simulink model "phase4_scheduler_application"  (R2026a)
settings: Solver=FixedStepDiscrete  EnableMultiTasking=on
undefined symbols (not defined in the file): CostWeights, MapMaximumNearestDistance, MapNormalizationMean, MapNormalizationScale, MapRawMaximum, MapRawMinimum, MapSafetyMargins, MapSampleTimes_s, MapX, MapY, MaximumCpuUtilization, MaximumHeadingError_rad, MaximumLateralError_m, ModeCpuAdmissible, ModeMeanCpuUtilization, phase4_scheduler_application
libraries: proctasklib x1
settings Model: Creator=The MathWorks, Inc.  LastModifiedBy=rayyu
settings SolverCC: PositivePriorityOrder=on
settings HardwareCC: ProdBitPerLong=64.0  ProdLargestAtomicInteger=LongLong  ProdLargestAtomicFloat=Double  ProdHWDeviceType=ARM Compatible->ARM Cortex-A (64-bit)  HardwareBoardFeatureSet=SoCBlockset
settings RTWCC: SystemTargetFile=ert.tlc  HardwareBoard=Xilinx Zynq UltraScale+ MPSoC ZCU102 Evaluation Kit  TLCOptions="-aInlineSetEventsForThisBaseRateFcn=TLC_FALSE -aSuppressMultiTaskScheduler=TLC_FALSE  -aRateBasedStepFcn=0"  GenerateReport=on  Toolchain=Linaro AArch64 Linux v6.3.1  IncludeHyperlinkInReport=on  LaunchReport=on  GenerateTraceInfo=on  GenerateTraceReport=on  GenerateTraceReportSl=on  GenerateTraceReportSf=on  GenerateTraceReportEml=on  Description=Embedded Coder
settings ERTTargetCC: ExtModeTransport=2.0  DynamicArrayContainerType=coder::array

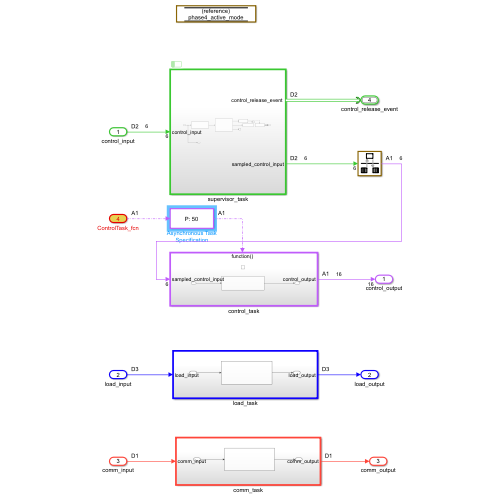
[thumbnail: Simulink's stored preview of the top-level diagram]
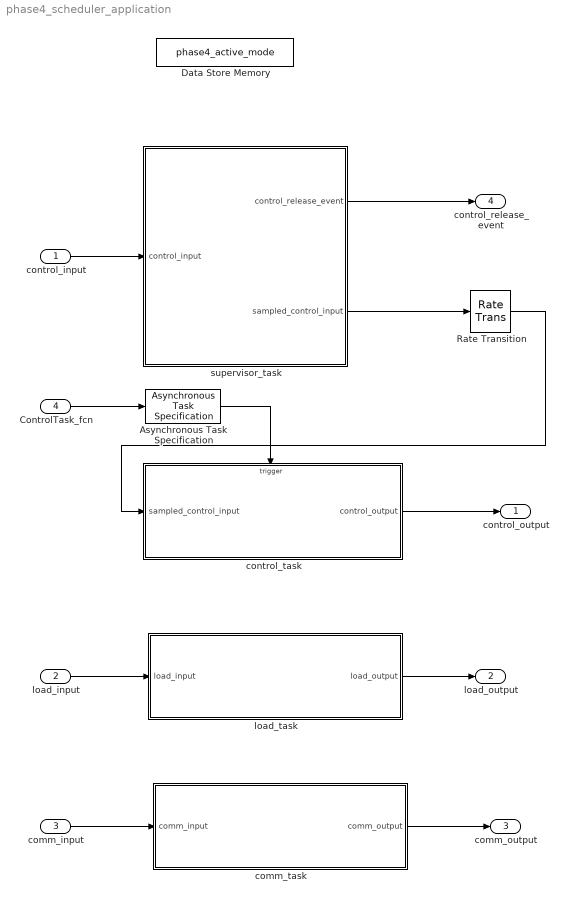
== system phase4_scheduler_application ==
  control_input : Inport
  load_input : Inport  Port=2  SampleTime=0.05  Interpolate=off
  comm_input : Inport  Port=3  SampleTime=0.005  Interpolate=off
  ControlTask_fcn : Inport  Port=4  OutputFunctionCall=on
  Asynchronous Task Specification : AsynchronousTaskSpecification  TaskPriority=50
  Data Store Memory : DataStoreMemory  DataStoreName=phase4_active_mode  WriteAfterWriteMsg=warning  DataStoreReference=on  ShowAdditionalParam=off  OutDataTypeStr=uint8  Dimensions=1
  Rate Transition : RateTransition  Deterministic=off
  comm_task : Subsystem  TreatAsAtomicUnit=on
  control_task : Subsystem  TreatAsAtomicUnit=on
  load_task : Subsystem  TreatAsAtomicUnit=on
  supervisor_task : Subsystem  TreatAsAtomicUnit=on  ScheduleAs=Periodic partition  PartitionName=SupervisorTask  SystemSampleTime=0.01
  control_output : Outport  VectorParamsAs1DForOutWhenUnconnected=off
  load_output : Outport  Port=2  VectorParamsAs1DForOutWhenUnconnected=off
  comm_output : Outport  Port=3
  control_release_event : Outport  InputPortMessageModes=m  Port=4  OutDataTypeStr=Bus: rteEvent  BusOutputAsStruct=on
  wires:
  control_task/1(control_output) -> control_output/1
  control_input/1 -> supervisor_task/1(control_input)
  load_input/1 -> load_task/1(load_input)
  load_task/1(load_output) -> load_output/1
  comm_input/1 -> comm_task/1(comm_input)
  comm_task/1(comm_output) -> comm_output/1
  supervisor_task/1("control_release_event ") -> control_release_event/1
  ControlTask_fcn/1 -> Asynchronous Task Specification/1
  Asynchronous Task Specification/1 -> control_task/Trigger
  supervisor_task/2(sampled_control_input) -> Rate Transition/1
  Rate Transition/1 -> control_task/1(sampled_control_input)

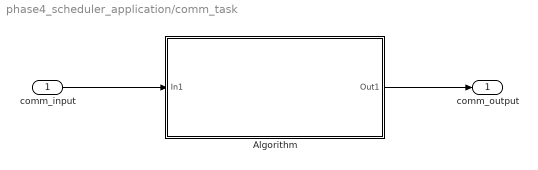
== system phase4_scheduler_application/comm_task ==
  comm_input : Inport
  Algorithm : Subsystem
  comm_output : Outport  VectorParamsAs1DForOutWhenUnconnected=off
  wires:
  comm_input/1 -> Algorithm/1(In1)
  Algorithm/1(Out1) -> comm_output/1

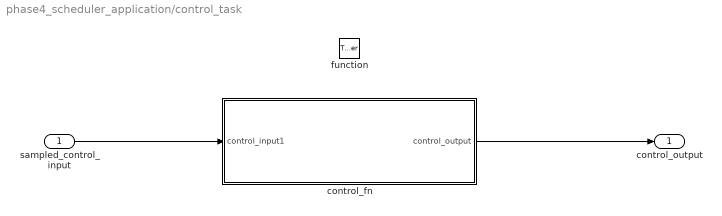
== system phase4_scheduler_application/control_task ==
  sampled_control_input : Inport
  function : TriggerPort  TriggerType=function-call  VariantControl=(inherit)
  control_fn : Subsystem  TreatAsAtomicUnit=on
  control_output : Outport
  wires:
  sampled_control_input/1 -> control_fn/1(control_input1)
  control_fn/1(control_output) -> control_output/1

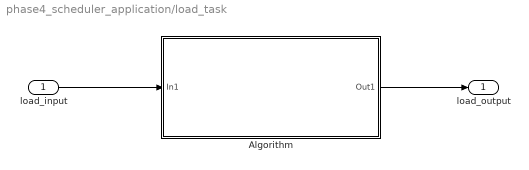
== system phase4_scheduler_application/load_task ==
  load_input : Inport
  Algorithm : Subsystem
  load_output : Outport  VectorParamsAs1DForOutWhenUnconnected=off
  wires:
  Algorithm/1(Out1) -> load_output/1
  load_input/1 -> Algorithm/1(In1)

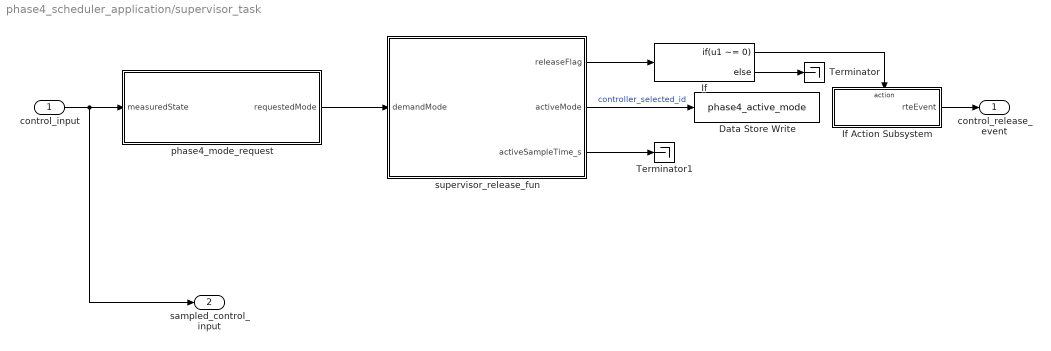
== system phase4_scheduler_application/supervisor_task ==
  control_input : Inport
  Data Store Write : DataStoreWrite  DataStoreName=phase4_active_mode  IndexOptions=Index vector (dialog)  Indices=1  OutputSizes=1
  If : If  IfExpression=u1 ~= 0
  If Action Subsystem : Subsystem  TreatAsAtomicUnit=on
  Terminator : Terminator
  Terminator1 : Terminator
  phase4_mode_request : Subsystem
  supervisor_release_fun : MATLAB Function  TreatAsAtomicUnit=on
  "control_release_event " : Outport  OutDataTypeStr=Bus: rteEvent
  sampled_control_input : Outport  Port=2
  wires:
  supervisor_release_fun/1(releaseFlag) -> If/1
  supervisor_release_fun/2(activeMode) -> Data Store Write/1  "controller_selected_id"
  supervisor_release_fun/3(activeSampleTime_s) -> Terminator1/1
  If/1 -> If Action Subsystem/Action
  If/2 -> Terminator/1
  If Action Subsystem/1(rteEvent) -> "control_release_event "/1
  phase4_mode_request/1(requestedMode) -> supervisor_release_fun/1(demandMode)
  control_input/1 -> sampled_control_input/1, phase4_mode_request/1(measuredState)

== system phase4_scheduler_application/comm_task/Algorithm ==
  In1 : Inport
  Gain : Gain  Gain=-1
  Out1 : Outport  VectorParamsAs1DForOutWhenUnconnected=off
  wires:
  Gain/1 -> Out1/1
  In1/1 -> Gain/1

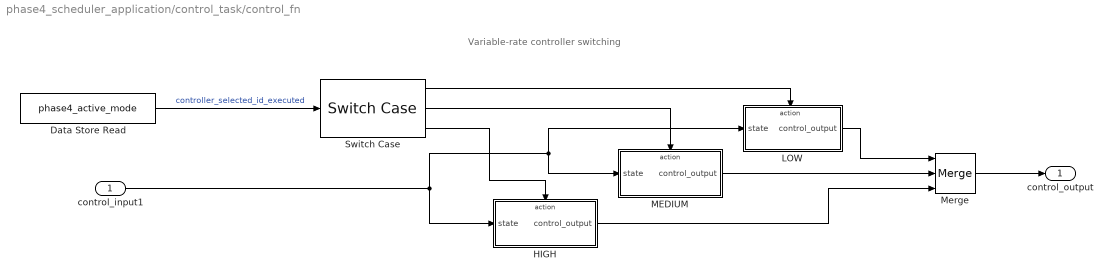
== system phase4_scheduler_application/control_task/control_fn ==
  note: Variable-rate controller switching
  control_input1 : Inport
  Data Store Read : DataStoreRead  DataStoreName=phase4_active_mode  IndexOptions=Index vector (dialog)  Indices=1  OutputSizes=1
  HIGH : Subsystem  TreatAsAtomicUnit=on
  LOW : Subsystem  TreatAsAtomicUnit=on
  MEDIUM : Subsystem  TreatAsAtomicUnit=on
  Merge : Merge  Inputs=3
  Switch Case : SwitchCase  CaseConditions={1, 2, 3}  ShowDefaultCase=off
  control_output : Outport
  wires:
  control_input1/1 -> HIGH/1(state), LOW/1(state), MEDIUM/1(state)
  Data Store Read/1 -> Switch Case/1  "controller_selected_id_executed"
  Switch Case/1 -> LOW/Action
  Switch Case/2 -> MEDIUM/Action
  Switch Case/3 -> HIGH/Action
  LOW/1(control_output) -> Merge/1
  MEDIUM/1(control_output) -> Merge/2
  HIGH/1(control_output) -> Merge/3
  Merge/1 -> control_output/1

== system phase4_scheduler_application/load_task/Algorithm ==
  In1 : Inport
  Gain : Gain  Gain=-1
  Out1 : Outport  VectorParamsAs1DForOutWhenUnconnected=off
  wires:
  In1/1 -> Gain/1
  Gain/1 -> Out1/1

== system phase4_scheduler_application/supervisor_task/If Action Subsystem ==
  Action Port : ActionPort  ActionPortLabel=if(u1 ~= 0)
  Task Trigger : proctasklib/Task Trigger  BlockSID=phase4_scheduler_application:90
  rteEvent : Outport
  wires:
  Task Trigger/1 -> rteEvent/1

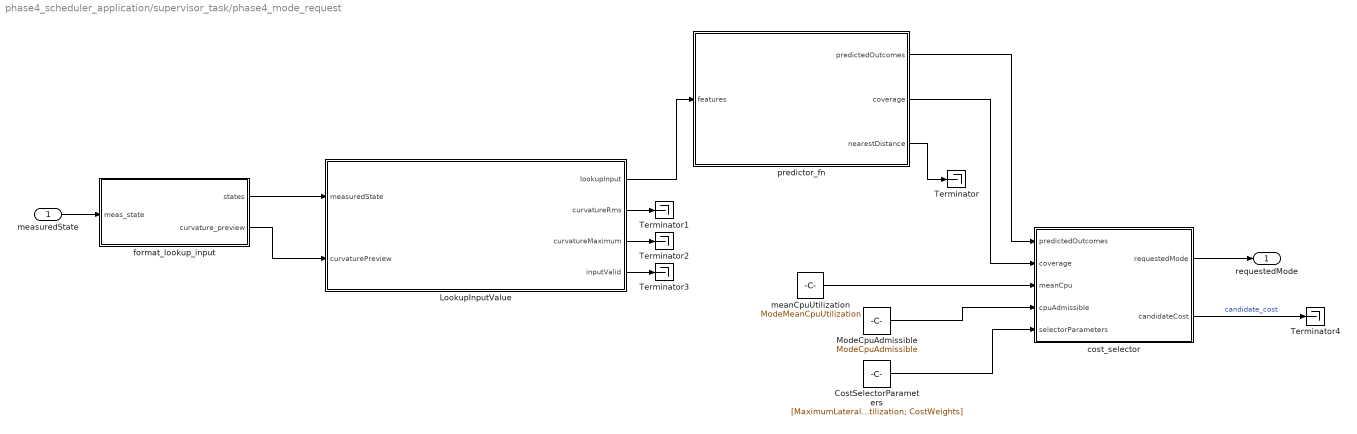
== system phase4_scheduler_application/supervisor_task/phase4_mode_request ==
  measuredState : Inport
  CostSelectorParameters : Constant  Value=[MaximumLateralError_m; MaximumHeadingError_rad; MaximumCpuUtilization; CostWeights]
  LookupInputValue : MATLAB Function  TreatAsAtomicUnit=on
  ModeCpuAdmissible : Constant  Value=ModeCpuAdmissible
  Terminator{,1..4} (5 alike) : Terminator
  cost_selector : MATLAB Function  TreatAsAtomicUnit=on
  format_lookup_input : Subsystem
  meanCpuUtilization : Constant  Value=ModeMeanCpuUtilization
  predictor_fn : MATLAB Function  TreatAsAtomicUnit=on
  requestedMode : Outport
  wires:
  LookupInputValue/1(lookupInput) -> predictor_fn/1(features)
  measuredState/1 -> format_lookup_input/1(meas_state)
  format_lookup_input/1(states) -> LookupInputValue/1(measuredState)
  format_lookup_input/2(curvature_preview) -> LookupInputValue/2(curvaturePreview)
  predictor_fn/1(predictedOutcomes) -> cost_selector/1(predictedOutcomes)
  predictor_fn/2(coverage) -> cost_selector/2(coverage)
  meanCpuUtilization/1 -> cost_selector/3(meanCpu)
  ModeCpuAdmissible/1 -> cost_selector/4(cpuAdmissible)
  CostSelectorParameters/1 -> cost_selector/5(selectorParameters)
  cost_selector/1(requestedMode) -> requestedMode/1
  predictor_fn/3(nearestDistance) -> Terminator/1
  LookupInputValue/2(curvatureRms) -> Terminator1/1
  LookupInputValue/3(curvatureMaximum) -> Terminator2/1
  LookupInputValue/4(inputValid) -> Terminator3/1
  cost_selector/2(candidateCost) -> Terminator4/1  "candidate_cost"

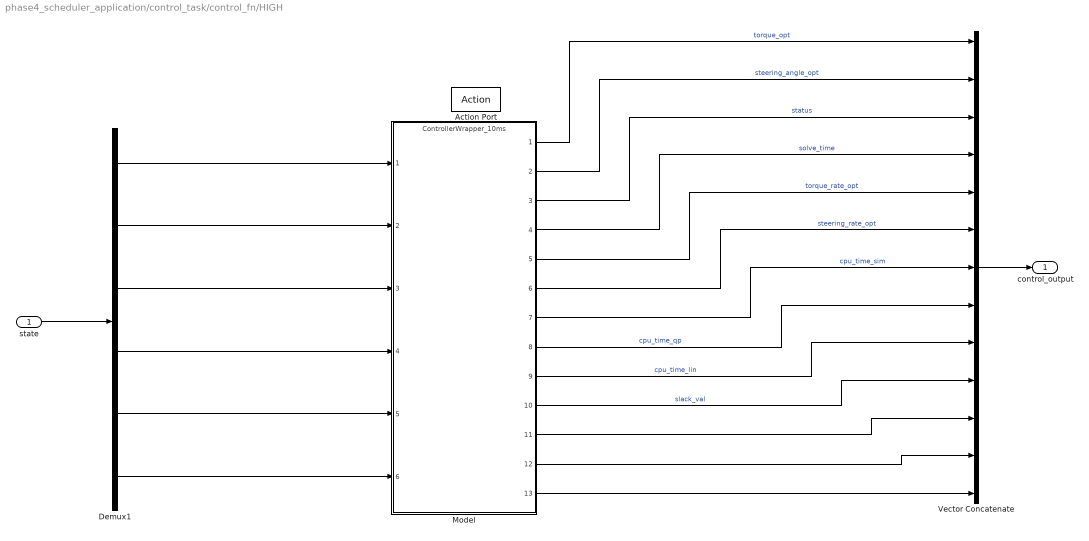
== system phase4_scheduler_application/control_task/control_fn/HIGH ==
  state : Inport
  Action Port : ActionPort  ActionPortLabel=case [ 3 ]:
  Demux1 : Demux  Outputs=6
  Model : ModelReference  ModelNameDialog=ControllerWrapper_10ms.slx  SimulationMode=Normal  ModelReferenceVersion=1.55
  Vector Concatenate : Concatenate  NumInputs=13
  control_output : Outport
  wires:
  Demux1/3 -> Model/3
  Demux1/2 -> Model/2
  Demux1/6 -> Model/6
  Demux1/1 -> Model/1
  state/1 -> Demux1/1
  Demux1/5 -> Model/5
  Demux1/4 -> Model/4
  Model/4 -> Vector Concatenate/4  "solve_time"
  Model/10 -> Vector Concatenate/10  "slack_val"
  Model/3 -> Vector Concatenate/3  "status"
  Model/8 -> Vector Concatenate/8  "cpu_time_qp"
  Model/1 -> Vector Concatenate/1  "torque_opt"
  Model/6 -> Vector Concatenate/6  "steering_rate_opt"
  Vector Concatenate/1 -> control_output/1
  Model/9 -> Vector Concatenate/9  "cpu_time_lin"
  Model/7 -> Vector Concatenate/7  "cpu_time_sim"
  Model/2 -> Vector Concatenate/2  "steering_angle_opt"
  Model/5 -> Vector Concatenate/5  "torque_rate_opt"
  Model/11 -> Vector Concatenate/11
  Model/12 -> Vector Concatenate/12
  Model/13 -> Vector Concatenate/13

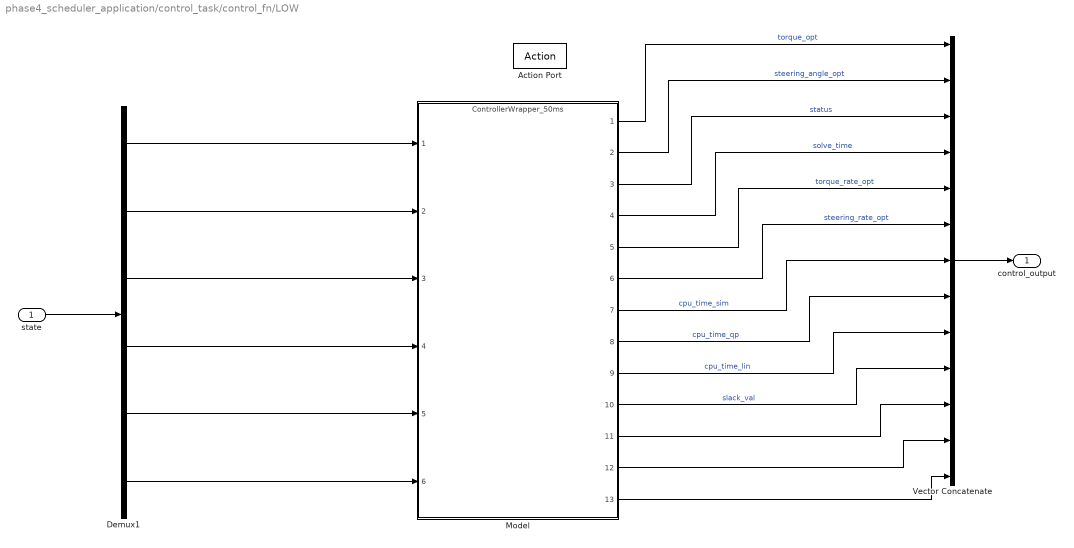
== system phase4_scheduler_application/control_task/control_fn/LOW ==
  state : Inport
  Action Port : ActionPort  ActionPortLabel=case [ 1 ]:
  Demux1 : Demux  Outputs=6
  Model : ModelReference  ModelNameDialog=ControllerWrapper_50ms.slx  SimulationMode=Normal  ModelReferenceVersion=1.51
  Vector Concatenate : Concatenate  NumInputs=13
  control_output : Outport
  wires:
  Demux1/3 -> Model/3
  Demux1/2 -> Model/2
  Demux1/6 -> Model/6
  Demux1/1 -> Model/1
  state/1 -> Demux1/1
  Demux1/5 -> Model/5
  Demux1/4 -> Model/4
  Model/4 -> Vector Concatenate/4  "solve_time"
  Model/10 -> Vector Concatenate/10  "slack_val"
  Model/3 -> Vector Concatenate/3  "status"
  Model/8 -> Vector Concatenate/8  "cpu_time_qp"
  Model/1 -> Vector Concatenate/1  "torque_opt"
  Model/6 -> Vector Concatenate/6  "steering_rate_opt"
  Vector Concatenate/1 -> control_output/1
  Model/9 -> Vector Concatenate/9  "cpu_time_lin"
  Model/7 -> Vector Concatenate/7  "cpu_time_sim"
  Model/2 -> Vector Concatenate/2  "steering_angle_opt"
  Model/5 -> Vector Concatenate/5  "torque_rate_opt"
  Model/11 -> Vector Concatenate/11
  Model/12 -> Vector Concatenate/12
  Model/13 -> Vector Concatenate/13

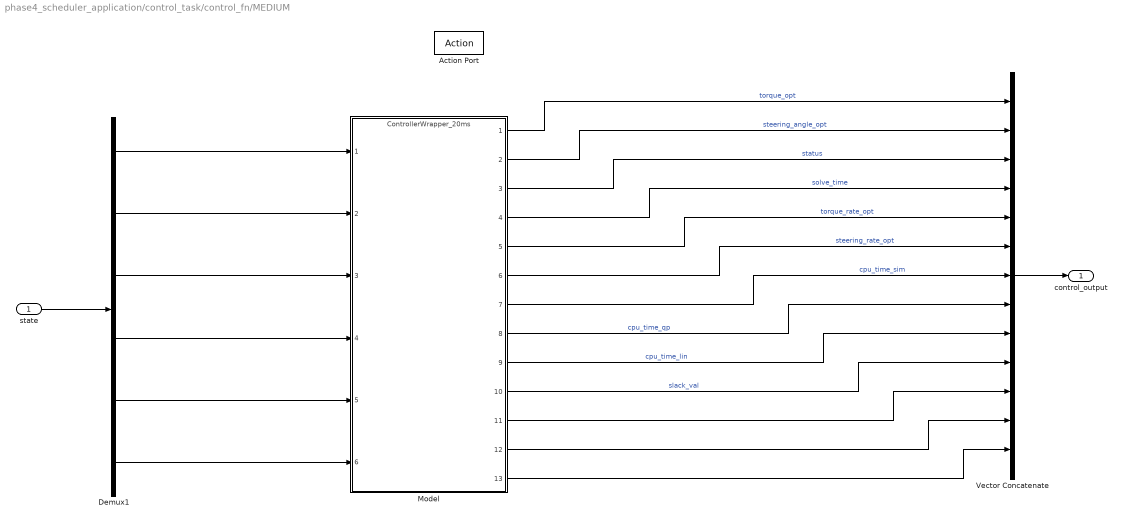
== system phase4_scheduler_application/control_task/control_fn/MEDIUM ==
  state : Inport
  Action Port : ActionPort  ActionPortLabel=case [ 2 ]:
  Demux1 : Demux  Outputs=6
  Model : ModelReference  ModelNameDialog=ControllerWrapper_20ms.slx  SimulationMode=Normal  ModelReferenceVersion=1.53
  Vector Concatenate : Concatenate  NumInputs=13
  control_output : Outport
  wires:
  Demux1/3 -> Model/3
  Demux1/2 -> Model/2
  Demux1/6 -> Model/6
  Demux1/1 -> Model/1
  state/1 -> Demux1/1
  Demux1/5 -> Model/5
  Demux1/4 -> Model/4
  Model/3 -> Vector Concatenate/3  "status"
  Model/4 -> Vector Concatenate/4  "solve_time"
  Model/2 -> Vector Concatenate/2  "steering_angle_opt"
  Model/1 -> Vector Concatenate/1  "torque_opt"
  Vector Concatenate/1 -> control_output/1
  Model/5 -> Vector Concatenate/5  "torque_rate_opt"
  Model/6 -> Vector Concatenate/6  "steering_rate_opt"
  Model/7 -> Vector Concatenate/7  "cpu_time_sim"
  Model/8 -> Vector Concatenate/8  "cpu_time_qp"
  Model/9 -> Vector Concatenate/9  "cpu_time_lin"
  Model/10 -> Vector Concatenate/10  "slack_val"
  Model/11 -> Vector Concatenate/11
  Model/12 -> Vector Concatenate/12
  Model/13 -> Vector Concatenate/13

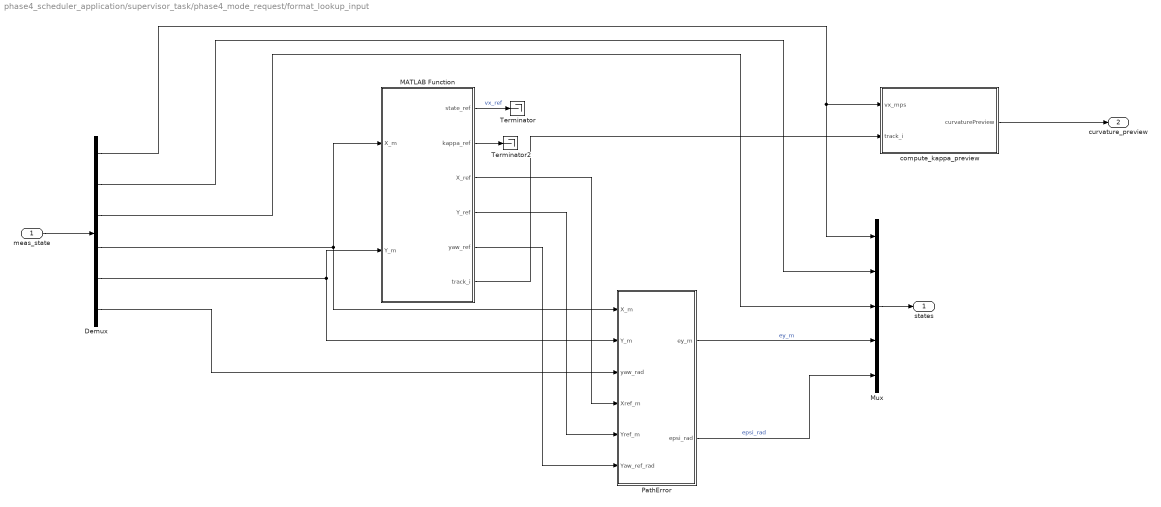
== system phase4_scheduler_application/supervisor_task/phase4_mode_request/format_lookup_input ==
  meas_state : Inport
  Demux : Demux  Outputs=6
  MATLAB Function : MATLAB Function  TreatAsAtomicUnit=on
  Mux : Mux  Inputs=5
  PathError : Subsystem
  Terminator : Terminator
  Terminator2 : Terminator
  compute_kappa_preview : MATLAB Function  TreatAsAtomicUnit=on
  states : Outport
  curvature_preview : Outport  Port=2
  wires:
  MATLAB Function/1(state_ref) -> Terminator/1  "vx_ref"
  MATLAB Function/2(kappa_ref) -> Terminator2/1
  MATLAB Function/3(X_ref) -> PathError/4(Xref_m)
  MATLAB Function/4(Y_ref) -> PathError/5(Yref_m)
  MATLAB Function/5(yaw_ref) -> PathError/6(Yaw_ref_rad)
  MATLAB Function/6(track_i) -> compute_kappa_preview/2(track_i)
  Demux/4 -> PathError/1(X_m), MATLAB Function/1(X_m)
  Demux/5 -> PathError/2(Y_m), MATLAB Function/2(Y_m)
  Demux/6 -> PathError/3(yaw_rad)
  PathError/1(ey_m) -> Mux/4  "ey_m"
  PathError/2(epsi_rad) -> Mux/5  "epsi_rad"
  meas_state/1 -> Demux/1
  Demux/1 -> Mux/1, compute_kappa_preview/1(vx_mps)
  Demux/2 -> Mux/2
  Demux/3 -> Mux/3
  Mux/1 -> states/1
  compute_kappa_preview/1(curvaturePreview) -> curvature_preview/1

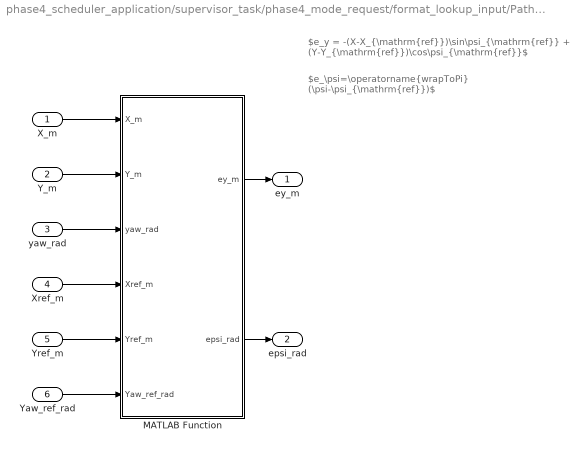
== system phase4_scheduler_application/supervisor_task/phase4_mode_request/format_lookup_input/PathError ==
  note: $e_\psi=\operatorname{wrapToPi} (\psi-\psi_{\mathrm{ref}})$
  note: $e_y = -(X-X_{\mathrm{ref}})\sin\psi_{\mathrm{ref}} + (Y-Y_{\mathrm{ref}})\cos\psi_{\mathrm{ref}}$
  X_m : Inport
  Y_m : Inport  Port=2
  yaw_rad : Inport  Port=3
  Xref_m : Inport  Port=4
  Yref_m : Inport  Port=5
  Yaw_ref_rad : Inport  Port=6
  MATLAB Function : MATLAB Function  TreatAsAtomicUnit=on
  ey_m : Outport
  epsi_rad : Outport  Port=2
  wires:
  X_m/1 -> MATLAB Function/1(X_m)
  Y_m/1 -> MATLAB Function/2(Y_m)
  yaw_rad/1 -> MATLAB Function/3(yaw_rad)
  Xref_m/1 -> MATLAB Function/4(Xref_m)
  Yref_m/1 -> MATLAB Function/5(Yref_m)
  Yaw_ref_rad/1 -> MATLAB Function/6(Yaw_ref_rad)
  MATLAB Function/1(ey_m) -> ey_m/1
  MATLAB Function/2(epsi_rad) -> epsi_rad/1

== matlab function phase4_scheduler_application/supervisor_task/phase4_mode_request/predictor_fn ==
  data: features input double size=[7 1]; predictedOutcomes output double size=[3 6]; coverage output boolean size=[3 1]; nearestDistance output double size=[3 1]; MapRawMaximum parameter size=[3 7]; MapX parameter size=[1146 7]; MapY parameter size=[1146 6]; MapSampleTimes_s parameter size=[1146 1]; MapNormalizationMean parameter size=[1 7]; MapNormalizationScale parameter size=[1 7]; MapRawMinimum parameter size=[3 7]; MapSafetyMargins parameter size=[1 6]; MapMaximumNearestDistance parameter size=[3 1]
function [predictedOutcomes, coverage, nearestDistance] = ...
    lookupPredictor(features, MapRawMaximum, MapX, MapY, MapSampleTimes_s, MapNormalizationMean, MapNormalizationScale, MapRawMinimum, MapSafetyMargins, MapMaximumNearestDistance)

candidateSampleTimes_s = [
    0.050
    0.020
    0.010
    ];

[predictedOutcomes, coverage, nearestDistance] = ...
    sdv.supervisor.predictFromLookupMap( ...
        features, ...
        candidateSampleTimes_s, ...
        MapX, ...
        MapY, ...
        MapSampleTimes_s, ...
        MapNormalizationMean, ...
        MapNormalizationScale, ...
        MapRawMinimum, ...
        MapRawMaximum, ...
        MapSafetyMargins, ...
        MapMaximumNearestDistance);
end

== matlab function phase4_scheduler_application/supervisor_task/supervisor_release_fun ==
  data: demandMode input; releaseFlag output; activeMode output; activeSampleTime_s output
function [ ...
    releaseFlag, ...
    activeMode, ...
    activeSampleTime_s] = ...
    supervisorReleaseLogic(demandMode)

persistent ticksRemaining
persistent latchedMode

if isempty(ticksRemaining)
    ticksRemaining = uint8(0);
    latchedMode = uint8(3);
end
%%MODE
% LOW = 1,     MEDIUM = 2,     HIGH = 3
% LOW = 50 ms, MEDIUM = 20 ms, HIGH = 10 ms.
periodTicks = uint8([5; 2; 1]); % number of ticks before it triggers the controller

requestedMode = uint8( ...
    min(max(double(demandMode), 1), 3));

% Escalate immediately when demand increases.
if requestedMode > latchedMode
    ticksRemaining = uint8(0); %% THIS WILL DROP THE CURRENT TASK AT THE MIDDLE OF EXECUTION TO START THE NEW SAMPLING RATE CONTROLLER
end

releaseFlag = ticksRemaining == 0; % release controller

if releaseFlag

    % Mode changes occur only at a controller release.
    latchedMode = requestedMode;

    ticksRemaining = ...
        periodTicks(double(latchedMode)) - uint8(1);

else
    ticksRemaining = ticksRemaining - uint8(1);
end

activeMode = latchedMode;

activeSampleTime_s = ...
    0.010 * double(periodTicks(double(activeMode)));

end

== matlab function phase4_scheduler_application/supervisor_task/phase4_mode_request/LookupInputValue ==
  data: measuredState input; lookupInput output; curvaturePreview input; curvatureRms output; curvatureMaximum output; inputValid output
function [ ...
    lookupInput, ...
    curvatureRms, ...
    curvatureMaximum, ...
    inputValid] = ...
    buildLookupInputValue( ...
        measuredState, ...
        curvaturePreview)

lookupInput = zeros(7, 1);
curvatureRms = 0;
curvatureMaximum = 0;

inputValid = ...
    all(isfinite(measuredState)) ...
    && all(isfinite(curvaturePreview));

if ~inputValid
    return;
end

vx_mps = measuredState(1);
vy_mps = measuredState(2);
yawRate_radps = measuredState(3);
ey_m = measuredState(4);
epsi_rad = measuredState(5);

numberOfPreviewPoints = ...
    numel(curvaturePreview);

curvatureRms = sqrt( ...
    sum(curvaturePreview.^2) ...
    / numberOfPreviewPoints);

curvatureMaximum = ...
    max(abs(curvaturePreview));

lookupInput = [
    abs(ey_m)
    abs(epsi_rad)
    vx_mps
    abs(vy_mps)
    abs(yawRate_radps)
    curvatureRms
    curvatureMaximum
    ];
end

== matlab function phase4_scheduler_application/supervisor_task/phase4_mode_request/format_lookup_input/MATLAB Function ==
  data: X_m input; state_ref output size=[1 5]; Y_m input; kappa_ref output; X_ref output; Y_ref output; yaw_ref output; track_ref_table parameter; track_i output
function [state_ref, ...
          kappa_ref, ...
          X_ref, ...
          Y_ref, ...
          yaw_ref, ...
          track_i ...
          ] = ...
          path_ref( ...
              X_m, ...
              Y_m,...
              track_ref_table)
% track_reference_table columns:
% 1: s
% 2: X
% 3: Y
% 4: psi
% 5: kappa
% 6: vx reference
% 7: yaw-rate reference

%% Find closest track point
distanceSquared = ...
    (track_ref_table(:,2) - X_m).^2 + ...
    (track_ref_table(:,3) - Y_m).^2;

[~, track_i] = min(distanceSquared);


%% Extract local path reference

X_ref = ...
    track_ref_table(track_i, 2);

Y_ref = ...
    track_ref_table(track_i, 3);

yaw_ref = ...
    track_ref_table(track_i, 4);

kappa_ref = ...
    track_ref_table(track_i, 5);

vx_reference = ...
    track_ref_table(track_i, 6);

yaw_rate_reference = ...
    track_ref_table(track_i, 7);

%% Construct MPC state reference

state_ref = zeros(1,5);

state_ref(1) = vx_reference;
state_ref(2) = 0;
state_ref(3) = yaw_rate_reference;
state_ref(4) = 0;
state_ref(5) = 0;

end

== matlab function phase4_scheduler_application/supervisor_task/phase4_mode_request/format_lookup_input/PathError/MATLAB Function ==
  data: X_m input; ey_m output; Y_m input; yaw_rad input; Xref_m input; Yref_m input; Yaw_ref_rad input; epsi_rad output
function [ey_m, epsi_rad] = ...
    PathError( ...
    X_m, ...
    Y_m, ...
    yaw_rad, ...
    Xref_m, ...
    Yref_m, ...
    Yaw_ref_rad)
% Position relative to the selected reference-path point
deltaX = X_m - Xref_m;
deltaY = Y_m - Yref_m;
% Signed lateral error
ey_m = ...
    -deltaX * sin(Yaw_ref_rad) + ...
    deltaY * cos(Yaw_ref_rad);
% Wrap heading error to [-pi, pi]
epsi_rad = atan2( ...
    sin(yaw_rad - Yaw_ref_rad), ...
    cos(yaw_rad - Yaw_ref_rad));

end

== matlab function phase4_scheduler_application/supervisor_task/phase4_mode_request/format_lookup_input/compute_kappa_preview ==
  data: vx_mps input; curvaturePreview output; track_i input; track_ref_table parameter double
function curvaturePreview = ...
    compute_kappa_preview(vx_mps, track_i, track_ref_table)
% Curvature preview over 1 second at 10 ms intervals.
%
% track_ref_table columns:
%   1 = station, m
%   5 = curvature, 1/m

numberOfIntervals = 100;
previewStep_s = 0.01;

curvaturePreview = zeros(101, 1);

numberOfTrackPoints = size(track_ref_table, 1);

currentIndex = round(track_i);
currentIndex = max(1, ...
    min(currentIndex, numberOfTrackPoints));

predictedStation_m = ...
    track_ref_table(currentIndex, 1);

curvaturePreview(1) = ...
    track_ref_table(currentIndex, 5);

previewSpeed_mps = max(vx_mps, 0);

for node = 2:(numberOfIntervals + 1)

    predictedStation_m = ...
        predictedStation_m ...
        + previewSpeed_mps * previewStep_s;

    while currentIndex < numberOfTrackPoints && ...
            track_ref_table(currentIndex, 1) ...
            < predictedStation_m

        currentIndex = currentIndex + 1;
    end

    curvaturePreview(node) = ...
        track_ref_table(currentIndex, 5);
end
end

== matlab function phase4_scheduler_application/supervisor_task/phase4_mode_request/cost_selector ==
  data: predictedOutcomes input double size=[3 6]; requestedMode output uint8 size=[1 1]; coverage input boolean; meanCpu input double size=[3 1]; cpuAdmissible input boolean size=[3 1]; selectorParameters input double size=[7 1]; candidateCost output
function [requestedMode, candidateCost] = costSelector( ...
        predictedOutcomes, coverage, meanCpu, ...
        cpuAdmissible, selectorParameters)

candidateSampleTimes_s = [
    0.050
    0.020
    0.010
    ];

costWeights = [
    selectorParameters(4)
    selectorParameters(5)
    selectorParameters(6)
    selectorParameters(7)
    ];

[requestedMode, candidateCost, ~] = ...
    sdv.supervisor.selectModeFromCost( ...
        predictedOutcomes, ...
        coverage, ...
        candidateSampleTimes_s, ...
        meanCpu, ...
        cpuAdmissible, ...
        selectorParameters(1), ...
        selectorParameters(2), ...
        selectorParameters(3), ...
        costWeights);
end
